simulink model "analysis_TW_UPFC"  (R2018a)
settings: Solver=FixedStepDiscrete  StartTime=0.0  StopTime=1.2  FixedStep=Ts  RelTol=1e-3
PreLoadFcn:
  | Ts=1/512/60;
undefined symbols (not defined in the file): DiscIntNeverNeededParam
libraries: powerlib x59, powerlib_meascontrol x31, simulink_extras x2, simulink x1
(part 2 of 7)

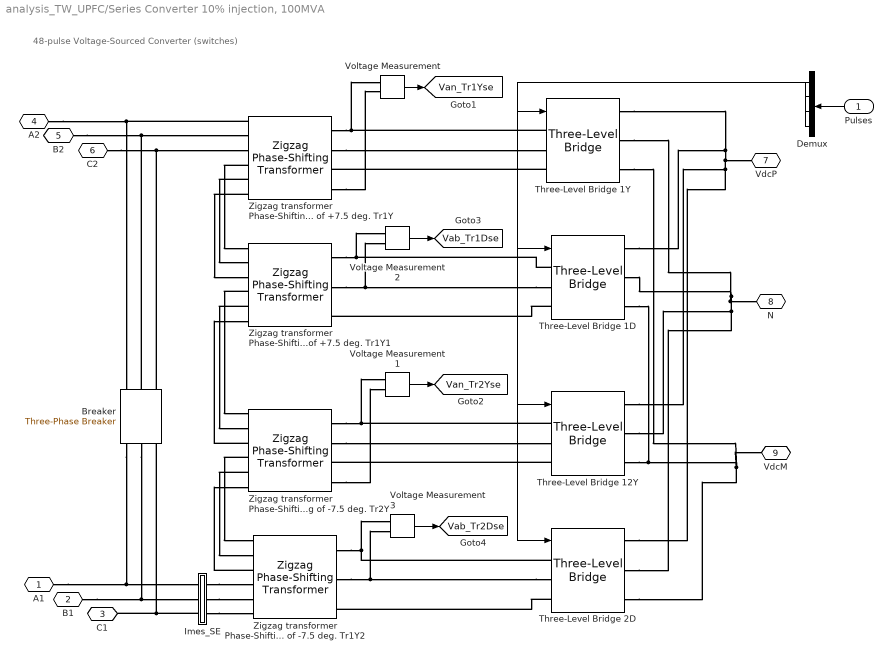
== system analysis_TW_UPFC/Series Converter 10% injection, 100MVA ==
  note: 48-pulse Voltage-Sourced Converter
      | (switches)
  Pulses : Inport  PortDimensions=48
  Breaker : powerlib/Elements/Three-Phase Breaker  InitialState=closed  SwitchA=on  SwitchB=on  SwitchC=on  SwitchTimes=[ 0]  External=off  BreakerResistance=0.0001  SnubberResistance=1e6  SnubberCapacitance=inf  Measurements=None
      settings: AttributesFormatString=\n
  Demux : Demux  Outputs=[12 12 12 12]
  Imes_SE : Subsystem
  Three-Level Bridge 12Y : powerlib/Power Electronics/Three-Level Bridge  Arms=3  SnubberResistance=1e5  SbubberCapacitance=inf  Device=GTO / Diodes  Ron=1e-4  ForwardVoltages="[  0  0  ]"  Measurements=None
      settings: SourceProductName=Simscape Power Systems  SourceProductBaseCode=PS
  Three-Level Bridge 1D : powerlib/Power Electronics/Three-Level Bridge  Arms=3  SnubberResistance=1e5  SbubberCapacitance=inf  Device=GTO / Diodes  Ron=1e-4  ForwardVoltages="[  0  0  ]"  Measurements=None
      settings: SourceProductName=Simscape Power Systems  SourceProductBaseCode=PS
  Three-Level Bridge 1Y : powerlib/Power Electronics/Three-Level Bridge  Arms=3  SnubberResistance=1e5  SbubberCapacitance=inf  Device=GTO / Diodes  Ron=1e-4  ForwardVoltages="[  0  0  ]"  Measurements=None
      settings: SourceProductName=Simscape Power Systems  SourceProductBaseCode=PS
  Three-Level Bridge 2D : powerlib/Power Electronics/Three-Level Bridge  Arms=3  SnubberResistance=1e5  SbubberCapacitance=inf  Device=GTO / Diodes  Ron=1e-4  ForwardVoltages="[  0  0  ]"  Measurements=None
      settings: SourceProductName=Simscape Power Systems  SourceProductBaseCode=PS
  Voltage Measurement{,1..3} (4 alike) : powerlib/Measurements/Voltage Measurement  Tag=PoWeRsYsTeMmEaSuReMeNt  PhasorSimulation=off  OutputType=Magnitude  PSBequivalent=0
  Zigzag transformer Phase-Shifting of +7.5 deg. Tr1Y : powerlib/Elements/Zigzag Phase-Shifting Transformer  SecondaryConnection=Yn  SetSaturation=off  SetInitialFlux=off  Measurements=None  UNITS=pu  NominalPower=[ 100e6/4 60]  PrimaryVoltage=12.5e3  SecondaryVoltage="[ 12.5e3  +7.5]"  Winding1=[ 0.05/30 0.05 ]  Winding2=[ 0.05/30 0.05 ]  Winding3=[ 0.05/30 0.05 ]  RmLm=[ 500 500 ]  Rm=500  Saturation=[ 0,0 ; 0.0024,1.2 ; 1.0,1.52 ]  InitialFluxes=[0,0,0]  MoreParameters=off  BreakLoop=off  DataType=off
      settings: AttributesFormatString=\n  SourceProductName=Simscape Power Systems  SourceProductBaseCode=PS
  Zigzag transformer Phase-Shifting of +7.5 deg. Tr1Y1 : powerlib/Elements/Zigzag Phase-Shifting Transformer  SecondaryConnection=Delta D1(-30 deg.)  SetSaturation=off  SetInitialFlux=off  Measurements=None  UNITS=pu  NominalPower=[ 100e6/4 60]  PrimaryVoltage=12.5e3  SecondaryVoltage="[ 12.5e3  +7.5]"  Winding1=[ 0.05/30 0.05 ]  Winding2=[ 0.05/30 0.05 ]  Winding3=[ 0.05/30 0.05 ]  RmLm=[ 500 500 ]  Rm=500  Saturation=[ 0,0 ; 0.0024,1.2 ; 1.0,1.52 ]  InitialFluxes=[0,0,0]  MoreParameters=off  BreakLoop=off  DataType=off
      settings: AttributesFormatString=\n  SourceProductName=Simscape Power Systems  SourceProductBaseCode=PS
  Zigzag transformer Phase-Shifting of -7.5 deg. Tr1Y2 : powerlib/Elements/Zigzag Phase-Shifting Transformer  SecondaryConnection=Delta D1(-30 deg.)  SetSaturation=off  SetInitialFlux=off  Measurements=None  UNITS=pu  NominalPower=[ 100e6/4 60]  PrimaryVoltage=12.5e3  SecondaryVoltage="[ 12.5e3  -7.5]"  Winding1=[ 0.05/30 0.05 ]  Winding2=[ 0.05/30 0.05 ]  Winding3=[ 0.05/30 0.05 ]  RmLm=[ 500 500 ]  Rm=500  Saturation=[ 0,0 ; 0.0024,1.2 ; 1.0,1.52 ]  InitialFluxes=[0,0,0]  MoreParameters=off  BreakLoop=off  DataType=off
      settings: AttributesFormatString=\n  SourceProductName=Simscape Power Systems  SourceProductBaseCode=PS
  Zigzag transformer Phase-Shifting of -7.5 deg. Tr2Y : powerlib/Elements/Zigzag Phase-Shifting Transformer  SecondaryConnection=Yn  SetSaturation=off  SetInitialFlux=off  Measurements=None  UNITS=pu  NominalPower=[ 100e6/4 60]  PrimaryVoltage=12.5e3  SecondaryVoltage="[ 12.5e3  -7.5]"  Winding1=[ 0.05/30 0.05 ]  Winding2=[ 0.05/30 0.05 ]  Winding3=[ 0.05/30 0.05 ]  RmLm=[ 500 500 ]  Rm=500  Saturation=[ 0,0 ; 0.0024,1.2 ; 1.0,1.52 ]  InitialFluxes=[0,0,0]  MoreParameters=off  BreakLoop=off  DataType=off
      settings: AttributesFormatString=\n  SourceProductName=Simscape Power Systems  SourceProductBaseCode=PS
  "A1 " : PMIOPort  Side=Left
  "B1 " : PMIOPort  Port=2  Side=Left
  C1 : PMIOPort  Port=3  Side=Left
  "A2 " : PMIOPort  Port=4  Side=Left
  "B2 " : PMIOPort  Port=5  Side=Left
  "C2 " : PMIOPort  Port=6  Side=Left
  VdcP : PMIOPort  Port=7  Side=Right
  N : PMIOPort  Port=8  Side=Right
  VdcM : PMIOPort  Port=9  Side=Right
  tag scope: Vab_Tr1Dse=global, Vab_Tr2Dse=global, Van_Tr1Yse=global, Van_Tr2Yse=global
  wires:
  Pulses/1 -> Demux/1
  Demux/4 -> Three-Level Bridge 2D/1
  Demux/3 -> Three-Level Bridge 12Y/1
  Demux/2 -> Three-Level Bridge 1D/1
  Demux/1 -> Three-Level Bridge 1Y/1
  Voltage Measurement3/1 -> [Vab_Tr2Dse]
  Voltage Measurement2/1 -> [Vab_Tr1Dse]
  Voltage Measurement1/1 -> [Van_Tr2Yse]
  Voltage Measurement/1 -> [Van_Tr1Yse]
  connections:
  Zigzag transformer Phase-Shifting of -7.5 deg. Tr2Y/RConn4 -- Voltage Measurement1/LConn2
  Zigzag transformer Phase-Shifting of +7.5 deg. Tr1Y/RConn4 -- Voltage Measurement/LConn2
  Three-Level Bridge 1Y/RConn3 -- Three-Level Bridge 1D/RConn3 -- Three-Level Bridge 12Y/RConn3 -- VdcM/RConn1 -- Three-Level Bridge 2D/RConn3
  Three-Level Bridge 12Y/RConn2 -- Three-Level Bridge 1D/RConn2 -- Three-Level Bridge 1Y/RConn2 -- N/RConn1 -- Three-Level Bridge 2D/RConn2
  Three-Level Bridge 1Y/RConn1 -- Three-Level Bridge 12Y/RConn1 -- Three-Level Bridge 2D/RConn1 -- VdcP/RConn1 -- Three-Level Bridge 1D/RConn1
  Three-Level Bridge 1D/LConn1 -- Zigzag transformer Phase-Shifting of +7.5 deg. Tr1Y1/RConn1 -- Voltage Measurement2/LConn1
  Imes_SE/RConn1 -- Zigzag transformer Phase-Shifting of -7.5 deg. Tr1Y2/LConn4
  Imes_SE/RConn2 -- Zigzag transformer Phase-Shifting of -7.5 deg. Tr1Y2/LConn5
  Imes_SE/RConn3 -- Zigzag transformer Phase-Shifting of -7.5 deg. Tr1Y2/LConn6
  "A1 "/RConn1 -- Imes_SE/LConn1 -- Breaker/RConn1
  Zigzag transformer Phase-Shifting of +7.5 deg. Tr1Y/LConn4 -- Zigzag transformer Phase-Shifting of +7.5 deg. Tr1Y1/LConn1
  Zigzag transformer Phase-Shifting of +7.5 deg. Tr1Y/LConn5 -- Zigzag transformer Phase-Shifting of +7.5 deg. Tr1Y1/LConn2
  Zigzag transformer Phase-Shifting of +7.5 deg. Tr1Y/LConn6 -- Zigzag transformer Phase-Shifting of +7.5 deg. Tr1Y1/LConn3
  Zigzag transformer Phase-Shifting of +7.5 deg. Tr1Y1/LConn4 -- Zigzag transformer Phase-Shifting of -7.5 deg. Tr2Y/LConn1
  Zigzag transformer Phase-Shifting of +7.5 deg. Tr1Y1/LConn5 -- Zigzag transformer Phase-Shifting of -7.5 deg. Tr2Y/LConn2
  Zigzag transformer Phase-Shifting of -7.5 deg. Tr2Y/LConn3 -- Zigzag transformer Phase-Shifting of +7.5 deg. Tr1Y1/LConn6
  Zigzag transformer Phase-Shifting of -7.5 deg. Tr2Y/LConn4 -- Zigzag transformer Phase-Shifting of -7.5 deg. Tr1Y2/LConn1
  Zigzag transformer Phase-Shifting of -7.5 deg. Tr2Y/LConn5 -- Zigzag transformer Phase-Shifting of -7.5 deg. Tr1Y2/LConn2
  Zigzag transformer Phase-Shifting of -7.5 deg. Tr1Y2/LConn3 -- Zigzag transformer Phase-Shifting of -7.5 deg. Tr2Y/LConn6
  Three-Level Bridge 1Y/LConn1 -- Zigzag transformer Phase-Shifting of +7.5 deg. Tr1Y/RConn1 -- Voltage Measurement/LConn1
  Three-Level Bridge 12Y/LConn1 -- Zigzag transformer Phase-Shifting of -7.5 deg. Tr2Y/RConn1 -- Voltage Measurement1/LConn1
  Three-Level Bridge 2D/LConn1 -- Zigzag transformer Phase-Shifting of -7.5 deg. Tr1Y2/RConn1 -- Voltage Measurement3/LConn1
  Imes_SE/LConn3 -- Breaker/RConn3 -- C1/RConn1
  "B1 "/RConn1 -- Imes_SE/LConn2 -- Breaker/RConn2
  Breaker/LConn3 -- Zigzag transformer Phase-Shifting of +7.5 deg. Tr1Y/LConn3 -- "C2 "/RConn1
  Breaker/LConn2 -- Zigzag transformer Phase-Shifting of +7.5 deg. Tr1Y/LConn2 -- "B2 "/RConn1
  Zigzag transformer Phase-Shifting of +7.5 deg. Tr1Y/LConn1 -- Breaker/LConn1 -- "A2 "/RConn1
  Three-Level Bridge 1Y/LConn3 -- Zigzag transformer Phase-Shifting of +7.5 deg. Tr1Y/RConn3
  Zigzag transformer Phase-Shifting of +7.5 deg. Tr1Y/RConn2 -- Three-Level Bridge 1Y/LConn2
  Three-Level Bridge 1D/LConn2 -- Zigzag transformer Phase-Shifting of +7.5 deg. Tr1Y1/RConn2 -- Voltage Measurement2/LConn2
  Three-Level Bridge 1D/LConn3 -- Zigzag transformer Phase-Shifting of +7.5 deg. Tr1Y1/RConn3
  Zigzag transformer Phase-Shifting of -7.5 deg. Tr2Y/RConn2 -- Three-Level Bridge 12Y/LConn2
  Three-Level Bridge 12Y/LConn3 -- Zigzag transformer Phase-Shifting of -7.5 deg. Tr2Y/RConn3
  Three-Level Bridge 2D/LConn2 -- Zigzag transformer Phase-Shifting of -7.5 deg. Tr1Y2/RConn2 -- Voltage Measurement3/LConn2
  Three-Level Bridge 2D/LConn3 -- Zigzag transformer Phase-Shifting of -7.5 deg. Tr1Y2/RConn3

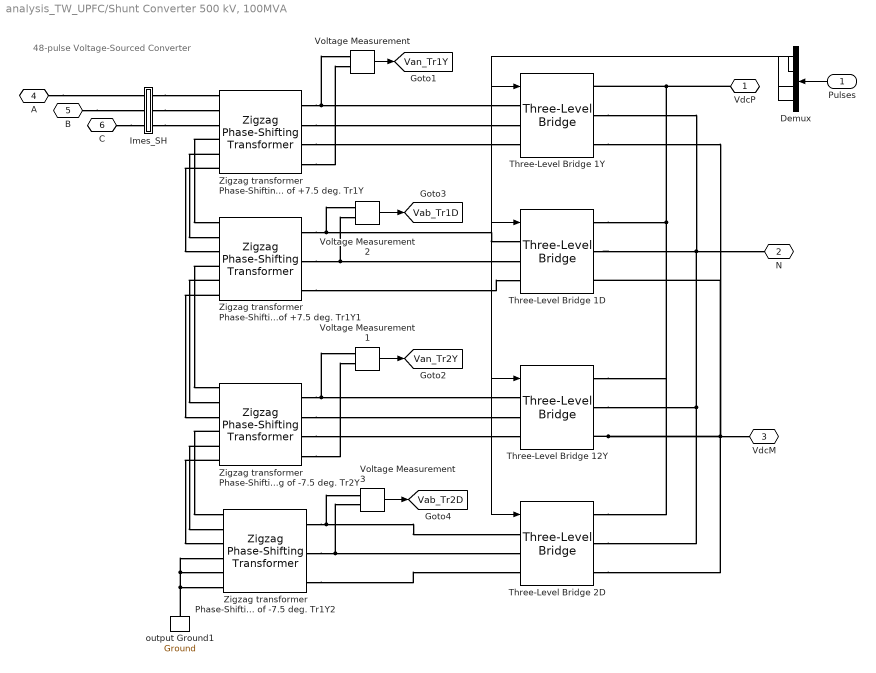
== system analysis_TW_UPFC/Shunt Converter 500 kV, 100MVA ==
  note: 48-pulse Voltage-Sourced Converter
  Pulses : Inport  PortDimensions=48
  Demux : Demux  Outputs=[12 12 12 12]
  Imes_SH : Subsystem
  Three-Level Bridge 12Y : powerlib/Power Electronics/Three-Level Bridge  Arms=3  SnubberResistance=1e5  SbubberCapacitance=inf  Device=GTO / Diodes  Ron=1e-4  ForwardVoltages="[  0  0  ]"  Measurements=None
      settings: SourceProductName=Simscape Power Systems  SourceProductBaseCode=PS
  Three-Level Bridge 1D : powerlib/Power Electronics/Three-Level Bridge  Arms=3  SnubberResistance=1e5  SbubberCapacitance=inf  Device=GTO / Diodes  Ron=1e-4  ForwardVoltages="[  0  0  ]"  Measurements=None
      settings: SourceProductName=Simscape Power Systems  SourceProductBaseCode=PS
  Three-Level Bridge 1Y : powerlib/Power Electronics/Three-Level Bridge  Arms=3  SnubberResistance=1e5  SbubberCapacitance=inf  Device=GTO / Diodes  Ron=1e-4  ForwardVoltages="[  0  0  ]"  Measurements=None
      settings: SourceProductName=Simscape Power Systems  SourceProductBaseCode=PS
  Three-Level Bridge 2D : powerlib/Power Electronics/Three-Level Bridge  Arms=3  SnubberResistance=1e5  SbubberCapacitance=inf  Device=GTO / Diodes  Ron=1e-4  ForwardVoltages="[  0  0  ]"  Measurements=None
      settings: SourceProductName=Simscape Power Systems  SourceProductBaseCode=PS
  Voltage Measurement{,1..3} (4 alike) : powerlib/Measurements/Voltage Measurement  Tag=PoWeRsYsTeMmEaSuReMeNt  PhasorSimulation=off  OutputType=Magnitude  PSBequivalent=0
  Zigzag transformer Phase-Shifting of +7.5 deg. Tr1Y : powerlib/Elements/Zigzag Phase-Shifting Transformer  SecondaryConnection=Yn  SetSaturation=off  SetInitialFlux=off  Measurements=None  UNITS=pu  NominalPower=[ 100e6/4 60]  PrimaryVoltage=500e3/4  SecondaryVoltage="[ 15e3  +7.5]"  Winding1=[ 0.05/30 0.05 ]  Winding2=[ 0.05/30 0.05 ]  Winding3=[ 0.05/30 0.05 ]  RmLm=[ 500 500 ]  Rm=500  Saturation=[ 0,0 ; 0.0024,1.2 ; 1.0,1.52 ]  InitialFluxes=[0,0,0]  MoreParameters=off  BreakLoop=off  DataType=off
      settings: AttributesFormatString=\n  SourceProductName=Simscape Power Systems  SourceProductBaseCode=PS
  Zigzag transformer Phase-Shifting of +7.5 deg. Tr1Y1 : powerlib/Elements/Zigzag Phase-Shifting Transformer  SecondaryConnection=Delta D1(-30 deg.)  SetSaturation=off  SetInitialFlux=off  Measurements=None  UNITS=pu  NominalPower=[ 100e6/4 60]  PrimaryVoltage=500e3/4  SecondaryVoltage="[ 15e3  +7.5]"  Winding1=[ 0.05/30 0.05 ]  Winding2=[ 0.05/30 0.05 ]  Winding3=[ 0.05/30 0.05 ]  RmLm=[ 500 500 ]  Rm=500  Saturation=[ 0,0 ; 0.0024,1.2 ; 1.0,1.52 ]  InitialFluxes=[0,0,0]  MoreParameters=off  BreakLoop=off  DataType=off
      settings: AttributesFormatString=\n  SourceProductName=Simscape Power Systems  SourceProductBaseCode=PS
  Zigzag transformer Phase-Shifting of -7.5 deg. Tr1Y2 : powerlib/Elements/Zigzag Phase-Shifting Transformer  SecondaryConnection=Delta D1(-30 deg.)  SetSaturation=off  SetInitialFlux=off  Measurements=None  UNITS=pu  NominalPower=[ 100e6/4 60]  PrimaryVoltage=500e3/4  SecondaryVoltage="[ 15e3  -7.5]"  Winding1=[ 0.05/30 0.05 ]  Winding2=[ 0.05/30 0.05 ]  Winding3=[ 0.05/30 0.05 ]  RmLm=[ 500 500 ]  Rm=500  Saturation=[ 0,0 ; 0.0024,1.2 ; 1.0,1.52 ]  InitialFluxes=[0,0,0]  MoreParameters=off  BreakLoop=off  DataType=off
      settings: AttributesFormatString=\n  SourceProductName=Simscape Power Systems  SourceProductBaseCode=PS
  Zigzag transformer Phase-Shifting of -7.5 deg. Tr2Y : powerlib/Elements/Zigzag Phase-Shifting Transformer  SecondaryConnection=Yn  SetSaturation=off  SetInitialFlux=off  Measurements=None  UNITS=pu  NominalPower=[ 100e6/4 60]  PrimaryVoltage=500e3/4  SecondaryVoltage="[ 15e3  -7.5]"  Winding1=[ 0.05/30 0.05 ]  Winding2=[ 0.05/30 0.05 ]  Winding3=[ 0.05/30 0.05 ]  RmLm=[ 500 500 ]  Rm=500  Saturation=[ 0,0 ; 0.0024,1.2 ; 1.0,1.52 ]  InitialFluxes=[0,0,0]  MoreParameters=off  BreakLoop=off  DataType=off
      settings: AttributesFormatString=\n  SourceProductName=Simscape Power Systems  SourceProductBaseCode=PS
  output Ground1 : powerlib/Elements/Ground  LConnTagsString=a  RConnTagsString=__newr0
  VdcP : PMIOPort  Side=Right
  N : PMIOPort  Port=2  Side=Right
  VdcM : PMIOPort  Port=3  Side=Right
  A : PMIOPort  Port=4  Side=Left
  B : PMIOPort  Port=5  Side=Left
  C : PMIOPort  Port=6  Side=Left
  tag scope: Vab_Tr1D=global, Vab_Tr2D=global, Van_Tr1Y=global, Van_Tr2Y=global
  wires:
  Pulses/1 -> Demux/1
  Voltage Measurement/1 -> [Van_Tr1Y]
  Voltage Measurement1/1 -> [Van_Tr2Y]
  Voltage Measurement2/1 -> [Vab_Tr1D]
  Voltage Measurement3/1 -> [Vab_Tr2D]
  Demux/1 -> Three-Level Bridge 1Y/1
  Demux/2 -> Three-Level Bridge 1D/1
  Demux/3 -> Three-Level Bridge 12Y/1
  Demux/4 -> Three-Level Bridge 2D/1
  connections:
  VdcP/RConn1 -- Three-Level Bridge 12Y/RConn1 -- Three-Level Bridge 2D/RConn1 -- Three-Level Bridge 1D/RConn1 -- Three-Level Bridge 1Y/RConn1
  Zigzag transformer Phase-Shifting of +7.5 deg. Tr1Y/RConn2 -- Three-Level Bridge 1Y/LConn2
  Zigzag transformer Phase-Shifting of +7.5 deg. Tr1Y/RConn3 -- Three-Level Bridge 1Y/LConn3
  Zigzag transformer Phase-Shifting of -7.5 deg. Tr2Y/RConn2 -- Three-Level Bridge 12Y/LConn2
  Zigzag transformer Phase-Shifting of -7.5 deg. Tr2Y/RConn3 -- Three-Level Bridge 12Y/LConn3
  Zigzag transformer Phase-Shifting of +7.5 deg. Tr1Y/RConn4 -- Voltage Measurement/LConn2
  Zigzag transformer Phase-Shifting of -7.5 deg. Tr2Y/RConn4 -- Voltage Measurement1/LConn2
  Imes_SH/RConn1 -- Zigzag transformer Phase-Shifting of +7.5 deg. Tr1Y/LConn1
  Imes_SH/RConn2 -- Zigzag transformer Phase-Shifting of +7.5 deg. Tr1Y/LConn2
  Imes_SH/RConn3 -- Zigzag transformer Phase-Shifting of +7.5 deg. Tr1Y/LConn3
  B/RConn1 -- Imes_SH/LConn2
  A/RConn1 -- Imes_SH/LConn1
  C/RConn1 -- Imes_SH/LConn3
  Zigzag transformer Phase-Shifting of +7.5 deg. Tr1Y/LConn4 -- Zigzag transformer Phase-Shifting of +7.5 deg. Tr1Y1/LConn1
  Zigzag transformer Phase-Shifting of +7.5 deg. Tr1Y/LConn5 -- Zigzag transformer Phase-Shifting of +7.5 deg. Tr1Y1/LConn2
  Zigzag transformer Phase-Shifting of +7.5 deg. Tr1Y/LConn6 -- Zigzag transformer Phase-Shifting of +7.5 deg. Tr1Y1/LConn3
  Zigzag transformer Phase-Shifting of +7.5 deg. Tr1Y1/LConn4 -- Zigzag transformer Phase-Shifting of -7.5 deg. Tr2Y/LConn1
  Zigzag transformer Phase-Shifting of +7.5 deg. Tr1Y1/LConn5 -- Zigzag transformer Phase-Shifting of -7.5 deg. Tr2Y/LConn2
  Zigzag transformer Phase-Shifting of +7.5 deg. Tr1Y1/LConn6 -- Zigzag transformer Phase-Shifting of -7.5 deg. Tr2Y/LConn3
  Zigzag transformer Phase-Shifting of -7.5 deg. Tr2Y/LConn4 -- Zigzag transformer Phase-Shifting of -7.5 deg. Tr1Y2/LConn1
  Zigzag transformer Phase-Shifting of -7.5 deg. Tr2Y/LConn5 -- Zigzag transformer Phase-Shifting of -7.5 deg. Tr1Y2/LConn2
  Zigzag transformer Phase-Shifting of -7.5 deg. Tr2Y/LConn6 -- Zigzag transformer Phase-Shifting of -7.5 deg. Tr1Y2/LConn3
  output Ground1/LConn1 -- Zigzag transformer Phase-Shifting of -7.5 deg. Tr1Y2/LConn4 -- Zigzag transformer Phase-Shifting of -7.5 deg. Tr1Y2/LConn5 -- Zigzag transformer Phase-Shifting of -7.5 deg. Tr1Y2/LConn6
  Three-Level Bridge 12Y/RConn3 -- Three-Level Bridge 1Y/RConn3 -- Three-Level Bridge 1D/RConn3 -- Three-Level Bridge 2D/RConn3 -- VdcM/RConn1
  Zigzag transformer Phase-Shifting of +7.5 deg. Tr1Y1/RConn1 -- Three-Level Bridge 1D/LConn1 -- Voltage Measurement2/LConn1
  Zigzag transformer Phase-Shifting of +7.5 deg. Tr1Y1/RConn2 -- Three-Level Bridge 1D/LConn2 -- Voltage Measurement2/LConn2
  Zigzag transformer Phase-Shifting of +7.5 deg. Tr1Y1/RConn3 -- Three-Level Bridge 1D/LConn3
  Three-Level Bridge 12Y/RConn2 -- Three-Level Bridge 1D/RConn2 -- N/RConn1 -- Three-Level Bridge 1Y/RConn2 -- Three-Level Bridge 2D/RConn2
  Zigzag transformer Phase-Shifting of +7.5 deg. Tr1Y/RConn1 -- Three-Level Bridge 1Y/LConn1 -- Voltage Measurement/LConn1
  Zigzag transformer Phase-Shifting of -7.5 deg. Tr2Y/RConn1 -- Three-Level Bridge 12Y/LConn1 -- Voltage Measurement1/LConn1
  Zigzag transformer Phase-Shifting of -7.5 deg. Tr1Y2/RConn1 -- Three-Level Bridge 2D/LConn1 -- Voltage Measurement3/LConn1
  Zigzag transformer Phase-Shifting of -7.5 deg. Tr1Y2/RConn2 -- Three-Level Bridge 2D/LConn2 -- Voltage Measurement3/LConn2
  Zigzag transformer Phase-Shifting of -7.5 deg. Tr1Y2/RConn3 -- Three-Level Bridge 2D/LConn3

== system analysis_TW_UPFC/Subsystem ==
  Sw1 : powerlib/Power Electronics/Ideal Switch  Ron=0.0001  Lon=0  IC=0  Rs=inf  Cs=0  Measurements=off
      settings: AttributesFormatString=\n
  Sw2 : powerlib/Power Electronics/Ideal Switch  Ron=0.0001  Lon=0  IC=0  Rs=inf  Cs=0  Measurements=off
      settings: AttributesFormatString=\n
  "VdcP " : PMIOPort  Side=Left
  "N " : PMIOPort  Port=2  Side=Left
  "VdcM " : PMIOPort  Port=3  Side=Left
  " VdcP" : PMIOPort  Port=4  Side=Right
  " N" : PMIOPort  Port=5  Side=Right
  " VdcM" : PMIOPort  Port=6  Side=Right
  wires:
  [Sw_On] -> Sw1/1, Sw2/1
  connections:
  " VdcP"/RConn1 -- Sw1/RConn1
  "VdcP "/RConn1 -- Sw1/LConn1
  " VdcM"/RConn1 -- Sw2/RConn1
  "VdcM "/RConn1 -- Sw2/LConn1
  "N "/RConn1 -- " N"/RConn1

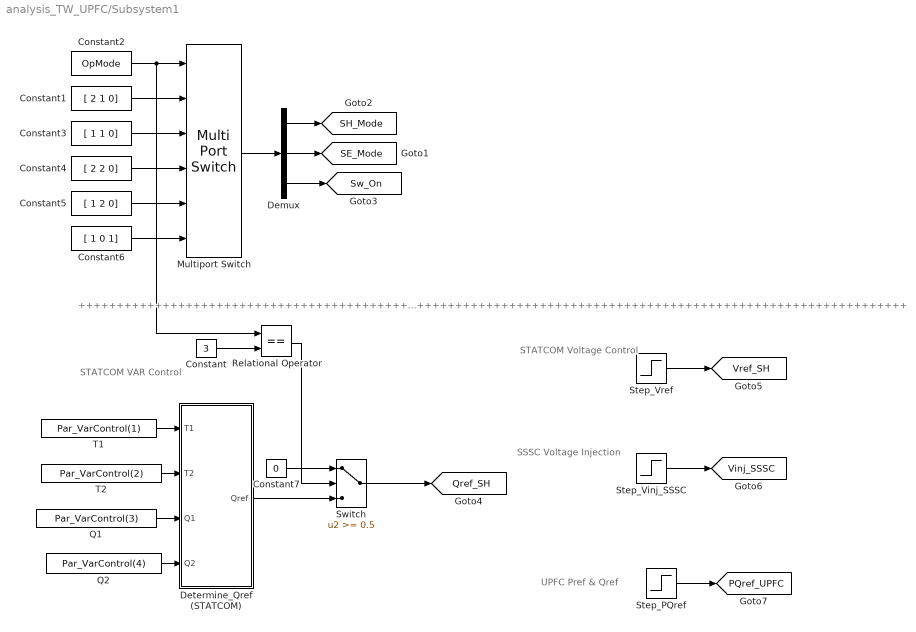
== system analysis_TW_UPFC/Subsystem1 ==
  note: +++++++++++++++++++++++++++++++++++++++++++++++++++++++++++++++++++++++++++++++++++++++++++++++++++++++++++++++++++
  note: STATCOM
      | VAR Control
  note: STATCOM
      | Voltage Control
  note: SSSC
      | Voltage Injection
  note: UPFC
      | Pref & Qref
  Constant : Constant  Value=3
  Constant1 : Constant  Value=[ 2 1 0]
  Constant2 : Constant  Value=OpMode
  Constant3 : Constant  Value=[ 1 1 0]
  Constant4 : Constant  Value=[ 2 2 0]
  Constant5 : Constant  Value=[ 1 2 0]
  Constant6 : Constant  Value=[ 1 0 1]
  Constant7 : Constant  Value=0
  Demux : Demux  Outputs=3
  Determine_Qref (STATCOM) : Subsystem
  Multiport Switch : MultiPortSwitch  Inputs=5  SaturateOnIntegerOverflow=on
  Q1 : Constant  Value=Par_VarControl(3)
  Q2 : Constant  Value=Par_VarControl(4)
  Relational Operator : RelationalOperator  Operator===  RndMeth=Nearest
  Step_PQref : Step  Time=[Par_UPFC_Pref(3) Par_UPFC_Qref(3) ]  Before=[Par_UPFC_Pref(1) Par_UPFC_Qref(1) ]  After=[Par_UPFC_Pref(2) Par_UPFC_Qref(2) ]  SampleTime=0
  Step_Vinj_SSSC : Step  Time=Par_SSSC(3)  Before=Par_SSSC(1)  After=Par_SSSC(2)  SampleTime=0
  Step_Vref : Step  Time=Par_Vref(3)  Before=Par_Vref(1)  After=Par_Vref(2)  SampleTime=0
  Switch : Switch  Threshold=0.5  SaturateOnIntegerOverflow=on
  T1 : Constant  Value=Par_VarControl(1)
  T2 : Constant  Value=Par_VarControl(2)
  tag scope: PQref_UPFC=global, Qref_SH=global, SE_Mode=global, SH_Mode=global, Sw_On=global, Vinj_SSSC=global, Vref_SH=global
  wires:
  Constant2/1 -> Multiport Switch/1, Relational Operator/1
  Multiport Switch/1 -> Demux/1
  Demux/1 -> [SH_Mode]
  Demux/2 -> [SE_Mode]
  Demux/3 -> [Sw_On]
  Constant1/1 -> Multiport Switch/2
  Constant6/1 -> Multiport Switch/6
  Constant5/1 -> Multiport Switch/5
  Constant3/1 -> Multiport Switch/3
  Constant4/1 -> Multiport Switch/4
  T1/1 -> Determine_Qref (STATCOM)/1(T1)
  T2/1 -> Determine_Qref (STATCOM)/2(T2)
  Q1/1 -> Determine_Qref (STATCOM)/3(Q1)
  Q2/1 -> Determine_Qref (STATCOM)/4(Q2)
  Determine_Qref (STATCOM)/1(Qref) -> Switch/3
  Switch/1 -> [Qref_SH]
  Constant/1 -> Relational Operator/2
  Relational Operator/1 -> Switch/2
  Constant7/1 -> Switch/1
  Step_Vref/1 -> [Vref_SH]
  Step_PQref/1 -> [PQref_UPFC]
  Step_Vinj_SSSC/1 -> [Vinj_SSSC]

== system analysis_TW_UPFC/Subsystem2 ==

== system analysis_TW_UPFC/Subsystem4 ==
  Data Acquisition : Subsystem
  Mux : Mux  Inputs=2
  SSSC : Scope  NumInputPorts=6
  STATCOM : Scope  NumInputPorts=4
  Selector : Selector  InputPortWidth=3  IndexOptions=Index vector (dialog)  Indices=2  OutputSizes=1
  Selector1 : Selector  InputPortWidth=3  IndexOptions=Index vector (dialog)  Indices=2  OutputSizes=1
  Selector2 : Selector  InputPortWidth=2  IndexOptions=Index vector (dialog)  Indices=1  OutputSizes=1
  UPFC : Scope  NumInputPorts=4
  tag scope: Display_PQ=global, Display_V1=global
  wires:
  Data Acquisition/1(VsVpI_SH) -> STATCOM/1  "Vs Vp Ip (pu)"
  Data Acquisition/2(Vdc_SH) -> STATCOM/2  "Vdc (V)"
  Data Acquisition/3(Q_Qref_SH) -> STATCOM/3  "Q Qref (pu)"
  Data Acquisition/4(VmeasVref_SH) -> STATCOM/4, Selector2/1  "Vmeas Vref (pu)"
  Data Acquisition/6(Iabc_SE) -> SSSC/2  "Iabc (pu)"
  Data Acquisition/5(Vinj_SE) -> SSSC/1  "Vinj (pu)"
  Data Acquisition/7(Vmeas_Vref_SSSC) -> SSSC/3  "Mag_Vinj  / Vref (pu)"
  Data Acquisition/8(Vdc_SE) -> SSSC/4  "Vdc"
  Data Acquisition/9(P_L123) -> UPFC/3, SSSC/5, Selector/1  "P L1 L2 L3 (MW)"
  Data Acquisition/10(Q_L123) -> UPFC/4, SSSC/6, Selector1/1  "Q L1 L2 L3 (Mvar)"
  Data Acquisition/11(P_Pref_SE) -> UPFC/1  "P Pref (pu)"
  Data Acquisition/12(Q_Qref_SE) -> UPFC/2  "Q Qref (pu)"
  Selector/1 -> Mux/1
  Selector1/1 -> Mux/2
  Mux/1 -> [Display_PQ]
  Selector2/1 -> [Display_V1]

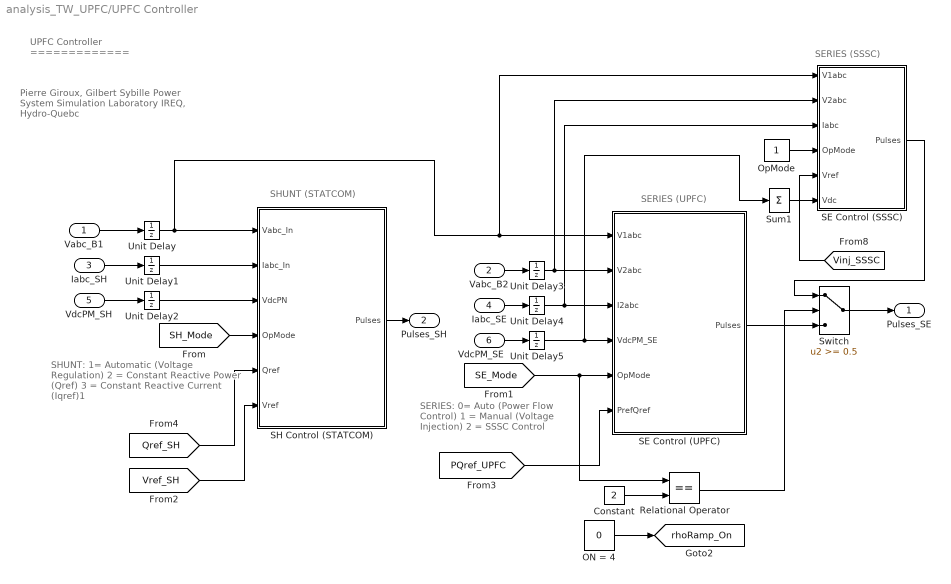
== system analysis_TW_UPFC/UPFC Controller ==
  note: Pierre Giroux, Gilbert Sybille
      | Power System Simulation Laboratory
      | IREQ, Hydro-Quebc
  note: SHUNT (STATCOM)
  note: SERIES (UPFC)
  note: UPFC Controller
      | =============
  note: SHUNT:
      | 1= Automatic (Voltage Regulation)
      | 2 = Constant Reactive Power (Qref)
      | 3 = Constant Reactive Current (Iqref)1
  note: SERIES:
      | 0= Auto (Power Flow Control)
      | 1 = Manual (Voltage Injection)
      | 2 = SSSC Control
  note: SERIES (SSSC)
  Vabc_B1 : Inport  PortDimensions=3
  Vabc_B2 : Inport  Port=2  PortDimensions=3
  "Iabc_SH " : Inport  Port=3  PortDimensions=3
  Iabc_SE : Inport  Port=4  PortDimensions=3
  "VdcPM_SH " : Inport  Port=5  PortDimensions=2
  VdcPM_SE : Inport  Port=6  PortDimensions=2
  Constant : Constant  Value=2
  ON = 4 : Constant  Value=0
  OpMode : Constant
  Relational Operator : RelationalOperator  Operator===  RndMeth=Nearest
  SE Control (SSSC) : Subsystem
  SE Control (UPFC) : Subsystem  mask(Injection Voltage Control){PQref=[8.7 -0.6], Vref_Inj=[0 0], ParK_Vseries=[0.045 1.5*4], Ts=Ts}
      mask prompts: PQref "Reference active and reactive power [ Pref  Qref ] (pu/100MVA):"; Vref_Inj "Manual Voltage Injection: [ Mag(pu)  rho(deg.) ]"; ParK_Vseries "Regulator gain [Kp  Ki ]"; Ts "Sample time:"
      mask init:
      | Kp_Vseries=ParK_Vseries(1);
      | Ki_Vseries=ParK_Vseries(2);
      | Pref=PQref(1);
      | Qref=PQref(2);
      | MagInj=Vref_Inj(1);
      | rhoInj=Vref_Inj(2);
  SH Control (STATCOM) : Subsystem  mask(STATCOM Controller){Vref=1.00, Droop=0.01, Qref1=0, Iqref1=0, ParK_V=[12 3000]*3, ParK_I=[5 40], Ts=Ts}
      mask prompts: Vref "Automatic mode: Voltage setpoint (Vref in pu)"; Droop "Droop (pu/100 MVA):"; Qref1 "Reactive power setpoint (Qref in pu)"; Iqref1 "Reactive Current setpoint (Iqref in pu):"; ParK_V "Voltage regulator gains: [ Kp  Ki ]"; ParK_I "Iq regulator gains: [ Kp  Ki ]"; Ts "Sample time:"
      mask init:
      | Kp_I=ParK_I(1);
      | Ki_I=ParK_I(2);
      | Kp_V=ParK_V(1);
      | Ki_V=ParK_V(2);
  Sum1 : Sum  Inputs=1  SaturateOnIntegerOverflow=on  InputSameDT=on  OutDataTypeStr=Inherit: Same as first input
  Switch : Switch  Threshold=0.5  SaturateOnIntegerOverflow=on
  Unit Delay{,1..5} (6 alike) : UnitDelay  SampleTime=Ts
  Pulses_SE : Outport
  Pulses_SH : Outport  Port=2
  tag scope: rhoRamp_On=global
  wires:
  "Iabc_SH "/1 -> Unit Delay1/1
  "VdcPM_SH "/1 -> Unit Delay2/1
  Vabc_B1/1 -> Unit Delay/1
  SH Control (STATCOM)/1(Pulses) -> Pulses_SH/1
  Iabc_SE/1 -> Unit Delay4/1
  Vabc_B2/1 -> Unit Delay3/1
  VdcPM_SE/1 -> Unit Delay5/1
  Unit Delay/1 -> SH Control (STATCOM)/1(Vabc_In), SE Control (UPFC)/1(V1abc), SE Control (SSSC)/1(V1abc)
  Unit Delay1/1 -> SH Control (STATCOM)/2(Iabc_In)
  Unit Delay2/1 -> SH Control (STATCOM)/3(VdcPN)
  Unit Delay3/1 -> SE Control (UPFC)/2(V2abc), SE Control (SSSC)/2(V2abc)
  Unit Delay4/1 -> SE Control (UPFC)/3(I2abc), SE Control (SSSC)/3(Iabc)
  Unit Delay5/1 -> SE Control (UPFC)/4(VdcPM_SE), Sum1/1
  ON = 4/1 -> [rhoRamp_On]
  [SE_Mode] -> SE Control (UPFC)/5(OpMode), Relational Operator/1
  OpMode/1 -> SE Control (SSSC)/4(OpMode)
  [SH_Mode] -> SH Control (STATCOM)/4(OpMode)
  Sum1/1 -> SE Control (SSSC)/6(Vdc)
  Constant/1 -> Relational Operator/2
  [Vref_SH] -> SH Control (STATCOM)/6(Vref)
  [PQref_UPFC] -> SE Control (UPFC)/6(PrefQref)
  [Vinj_SSSC] -> SE Control (SSSC)/5(Vref)
  [Qref_SH] -> SH Control (STATCOM)/5(Qref)
  SE Control (UPFC)/1(Pulses) -> Switch/3
  Switch/1 -> Pulses_SE/1
  SE Control (SSSC)/1(Pulses) -> Switch/1
  Relational Operator/1 -> Switch/2

== system analysis_TW_UPFC/info ==

== system analysis_TW_UPFC/Series Converter 10% injection, 100MVA/Imes_SE ==
  A->pu : Gain  Gain=500e3*sqrt(3)/100e6/sqrt(2)  SaturateOnIntegerOverflow=on  OutDataTypeStr=Inherit: Same as input  ParamDataTypeStr=Inherit: Same as input
  Current Measurement : powerlib/Measurements/Current Measurement  Tag=PoWeRsYsTeMmEaSuReMeNt  PhasorSimulation=off  OutputType=Magnitude  PSBequivalent=0
  Current Measurement1 : powerlib/Measurements/Current Measurement  Tag=PoWeRsYsTeMmEaSuReMeNt  PhasorSimulation=off  OutputType=Magnitude  PSBequivalent=0
  Current Measurement2 : powerlib/Measurements/Current Measurement  Tag=PoWeRsYsTeMmEaSuReMeNt  PhasorSimulation=off  OutputType=Magnitude  PSBequivalent=0
  Mux : Mux  Inputs=3
  "A " : PMIOPort  Side=Left
  "B " : PMIOPort  Port=2  Side=Left
  "C " : PMIOPort  Port=3  Side=Left
  " A" : PMIOPort  Port=4  Side=Right
  " B" : PMIOPort  Port=5  Side=Right
  " C" : PMIOPort  Port=6  Side=Right
  tag scope: Iabc_SE=global
  wires:
  Mux/1 -> A->pu/1
  A->pu/1 -> [Iabc_SE]
  Current Measurement/1 -> Mux/1
  Current Measurement2/1 -> Mux/3
  Current Measurement1/1 -> Mux/2
  connections:
  "A "/RConn1 -- Current Measurement/LConn1
  Current Measurement/RConn1 -- " A"/RConn1
  "B "/RConn1 -- Current Measurement1/LConn1
  Current Measurement1/RConn1 -- " B"/RConn1
  "C "/RConn1 -- Current Measurement2/LConn1
  Current Measurement2/RConn1 -- " C"/RConn1

== system analysis_TW_UPFC/Shunt Converter 500 kV, 100MVA/Imes_SH ==
  A->pu : Gain  Gain=500e3*sqrt(3)/100e6/sqrt(2)  SaturateOnIntegerOverflow=on  OutDataTypeStr=Inherit: Same as input  ParamDataTypeStr=Inherit: Same as input
  Current Measurement : powerlib/Measurements/Current Measurement  Tag=PoWeRsYsTeMmEaSuReMeNt  PhasorSimulation=off  OutputType=Magnitude  PSBequivalent=0
  Current Measurement1 : powerlib/Measurements/Current Measurement  Tag=PoWeRsYsTeMmEaSuReMeNt  PhasorSimulation=off  OutputType=Magnitude  PSBequivalent=0
  Current Measurement2 : powerlib/Measurements/Current Measurement  Tag=PoWeRsYsTeMmEaSuReMeNt  PhasorSimulation=off  OutputType=Magnitude  PSBequivalent=0
  Mux : Mux  Inputs=3
  "A " : PMIOPort  Side=Left
  "B " : PMIOPort  Port=2  Side=Left
  "C " : PMIOPort  Port=3  Side=Left
  " A" : PMIOPort  Port=4  Side=Right
  " B" : PMIOPort  Port=5  Side=Right
  " C" : PMIOPort  Port=6  Side=Right
  tag scope: Iabc_SH=global
  wires:
  Mux/1 -> A->pu/1
  A->pu/1 -> [Iabc_SH]
  Current Measurement/1 -> Mux/1
  Current Measurement2/1 -> Mux/3
  Current Measurement1/1 -> Mux/2
  connections:
  "A "/RConn1 -- Current Measurement/LConn1
  Current Measurement/RConn1 -- " A"/RConn1
  "B "/RConn1 -- Current Measurement1/LConn1
  Current Measurement1/RConn1 -- " B"/RConn1
  "C "/RConn1 -- Current Measurement2/LConn1
  Current Measurement2/RConn1 -- " C"/RConn1

== system analysis_TW_UPFC/Subsystem1/Determine_Qref (STATCOM) ==
  T1 : Inport
  T2 : Inport  Port=2
  Q1 : Inport  Port=3
  Q2 : Inport  Port=4
  Constant : Constant  Value=0
  Constant1 : Constant
  Digital Clock : DigitalClock  SampleTime=Ts
  Multiport Switch : MultiPortSwitch  SaturateOnIntegerOverflow=on
  Relational Operator : RelationalOperator  Operator=>  RndMeth=Nearest
  Relational Operator1 : RelationalOperator  Operator=>  RndMeth=Nearest
  Sum : Sum  Inputs=+++  SaturateOnIntegerOverflow=on
  Qref : Outport
  wires:
  Sum/1 -> Multiport Switch/1
  Q2/1 -> Multiport Switch/4
  Q1/1 -> Multiport Switch/3
  Multiport Switch/1 -> Qref/1
  Constant1/1 -> Sum/1
  Relational Operator1/1 -> Sum/3
  Relational Operator/1 -> Sum/2
  Constant/1 -> Multiport Switch/2
  T2/1 -> Relational Operator1/2
  T1/1 -> Relational Operator/2
  Digital Clock/1 -> Relational Operator1/1, Relational Operator/1

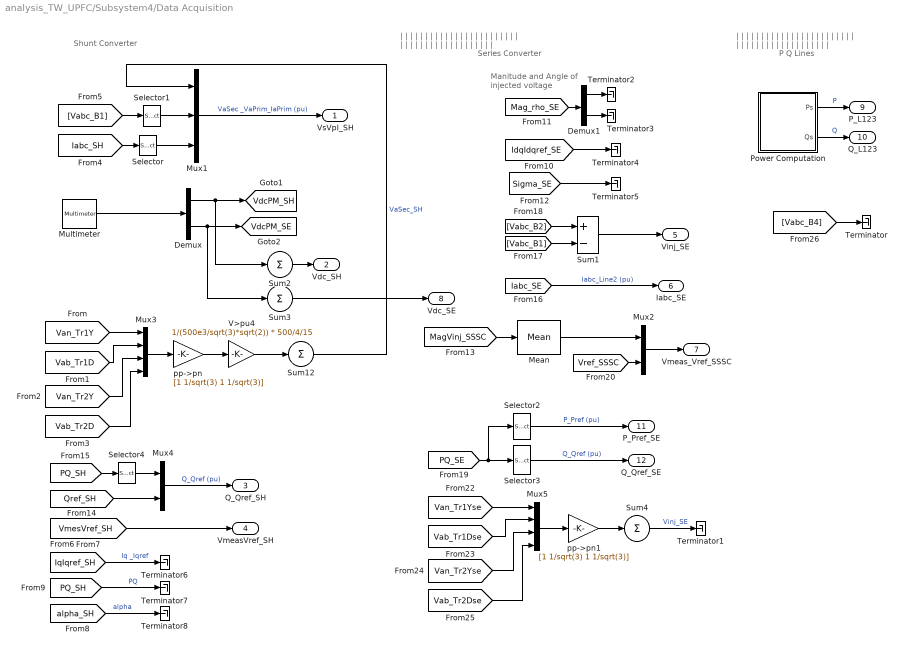
== system analysis_TW_UPFC/Subsystem4/Data Acquisition ==
  note: |
      | |
      | |
      | |
      | |
      | |
      | |
      | |
      | |
      | |
      | |
      | |
      | |
      | |
      | |
      | |
      | |
      | |
      | |
      | |
      | |
      | |
      | |
      | |
      | |
      | |
      | |
      | |
      | |
      | |
      | |
      | |
      | |
      | |
      | |
      | |
      | |
      | |
      | |
      | |
      | |
      | |
      | |
  note: Shunt Converter
  note: Series Converter
  note: |
      | |
      | |
      | |
      | |
      | |
      | |
      | |
      | |
      | |
      | |
      | |
      | |
      | |
      | |
      | |
      | |
      | |
      | |
      | |
      | |
      | |
      | |
      | |
      | |
      | |
      | |
      | |
      | |
      | |
      | |
      | |
      | |
      | |
      | |
      | |
      | |
      | |
      | |
      | |
      | |
      | |
      | |
  note: P Q Lines
  note: Manitude and Angle
      | of injected voltage
  Demux : Demux  Outputs=[2 2]
  Demux1 : Demux  Outputs=2
  Mean : powerlib_meascontrol/Measurements/Mean  Freq=60  Vinit=0  Ts=Ts
  Multimeter : powerlib/Measurements/Multimeter  Tag=PoWeRsYsTeMmEaSuReMeNt  PhasorSimulation=off  OutputType=Magnitude  sel=[4 2 3 1]  L=4  Gain=[1 1 1 1]  yselected={'Ub: Cp_SH','Ub: Cm_SH','Ub: Cp_SE','Ub: Cm_SE'};  PSBOutputType=1  PSBequivalent=0  AxesSetting=[0,0.1,-100,100]  Display=0  SavedBlockNames={}
      settings: AttributesFormatString=\n
  Mux1 : Mux  Inputs=3
  Mux2 : Mux  Inputs=2
  Mux3 : Mux
  Mux4 : Mux  Inputs=2
  Mux5 : Mux
  Power Computation : Subsystem
  Selector : Selector  InputPortWidth=3  IndexOptions=Index vector (dialog)  Indices=1  OutputSizes=1
  Selector1 : Selector  InputPortWidth=3  IndexOptions=Index vector (dialog)  Indices=1  OutputSizes=1
  Selector2 : Selector  InputPortWidth=4  IndexOptions=Index vector (dialog)  Indices=[1 3]  OutputSizes=1
  Selector3 : Selector  InputPortWidth=4  IndexOptions=Index vector (dialog)  Indices=[2 4]  OutputSizes=1
  Selector4 : Selector  InputPortWidth=2  IndexOptions=Index vector (dialog)  Indices=2  OutputSizes=1
  Sum1 : Sum  Inputs=+-  SaturateOnIntegerOverflow=on  InputSameDT=on  OutDataTypeStr=Inherit: Same as first input
  Sum{2..4,12} (4 alike) : Sum  Inputs=1  SaturateOnIntegerOverflow=on  InputSameDT=on  OutDataTypeStr=Inherit: Same as first input
  Terminator{,1..8} (9 alike) : Terminator
  V>pu4 : Gain  Gain=1/(500e3/sqrt(3)*sqrt(2)) * 500/4/15  SaturateOnIntegerOverflow=on  OutDataTypeStr=Inherit: Same as input  ParamDataTypeStr=Inherit: Same as input
  pp->pn : Gain  Gain=[1 1/sqrt(3) 1 1/sqrt(3)]  SaturateOnIntegerOverflow=on  OutDataTypeStr=Inherit: Same as input  ParamDataTypeStr=Inherit: Same as input
  pp->pn1 : Gain  Gain=[1 1/sqrt(3) 1 1/sqrt(3)]  SaturateOnIntegerOverflow=on  OutDataTypeStr=Inherit: Same as input  ParamDataTypeStr=Inherit: Same as input
  VsVpI_SH : Outport
  Vdc_SH : Outport  Port=2
  Q_Qref_SH : Outport  Port=3
  VmeasVref_SH : Outport  Port=4
  Vinj_SE : Outport  Port=5
  Iabc_SE : Outport  Port=6
  Vmeas_Vref_SSSC : Outport  Port=7
  Vdc_SE : Outport  Port=8
  P_L123 : Outport  Port=9
  Q_L123 : Outport  Port=10
  P_Pref_SE : Outport  Port=11
  Q_Qref_SE : Outport  Port=12
  tag scope: VdcPM_SE=global, VdcPM_SH=global
  wires:
  [Vref_SSSC] -> Mux2/2
  Mux2/1 -> Vmeas_Vref_SSSC/1
  [alpha_SH] -> Terminator8/1  "alpha"
  [PQ_SH] -> Terminator7/1  "PQ"
  [IqIqref_SH] -> Terminator6/1  "Iq _Iqref"
  [VmesVref_SH] -> VmeasVref_SH/1
  Selector3/1 -> Q_Qref_SE/1  "Q_Qref (pu)"
  [Sigma_SE] -> Terminator5/1
  [IdqIdqref_SE] -> Terminator4/1
  Demux1/2 -> Terminator3/1
  Demux1/1 -> Terminator2/1
  Sum4/1 -> Terminator1/1  "Vinj_SE"
  [Vabc_B4] -> Terminator/1
  [Iabc_SE] -> Iabc_SE/1  "Iabc_Line2 (pu)"
  Sum1/1 -> Vinj_SE/1
  Power Computation/2(Qs) -> Q_L123/1  "Q"
  Power Computation/1(Ps) -> P_L123/1  "P"
  [PQ_SE] -> Selector2/1, Selector3/1
  [Vabc_B1] -> Sum1/2
  [Vabc_B2] -> Sum1/1
  Selector2/1 -> P_Pref_SE/1  "P_Pref (pu)"
  [PQ_SH] -> Selector4/1
  Mux4/1 -> Q_Qref_SH/1  "Q_Qref (pu)"
  Selector4/1 -> Mux4/1
  [Qref_SH] -> Mux4/2
  V>pu4/1 -> Sum12/1
  pp->pn/1 -> V>pu4/1
  Mux3/1 -> pp->pn/1
  [Van_Tr1Y] -> Mux3/1
  [Vab_Tr1D] -> Mux3/2
  [Van_Tr2Y] -> Mux3/3
  [Vab_Tr2D] -> Mux3/4
  Mux1/1 -> VsVpI_SH/1  "VaSec _VaPrim_IaPrim (pu)"
  [Iabc_SH] -> Selector/1
  [Vabc_B1] -> Selector1/1
  Selector1/1 -> Mux1/2
  Selector/1 -> Mux1/3
  Sum12/1 -> Mux1/1  "VaSec_SH"
  Demux/1 -> [VdcPM_SH], Sum2/1
  Demux/2 -> [VdcPM_SE], Sum3/1
  Sum2/1 -> Vdc_SH/1
  Sum3/1 -> Vdc_SE/1
  pp->pn1/1 -> Sum4/1
  Mux5/1 -> pp->pn1/1
  [Van_Tr1Yse] -> Mux5/1
  [Vab_Tr1Dse] -> Mux5/2
  [Van_Tr2Yse] -> Mux5/3
  [Vab_Tr2Dse] -> Mux5/4
  [Mag_rho_SE] -> Demux1/1
  Multimeter/1 -> Demux/1
  [MagVinj_SSSC] -> Mean/1
  Mean/1 -> Mux2/1

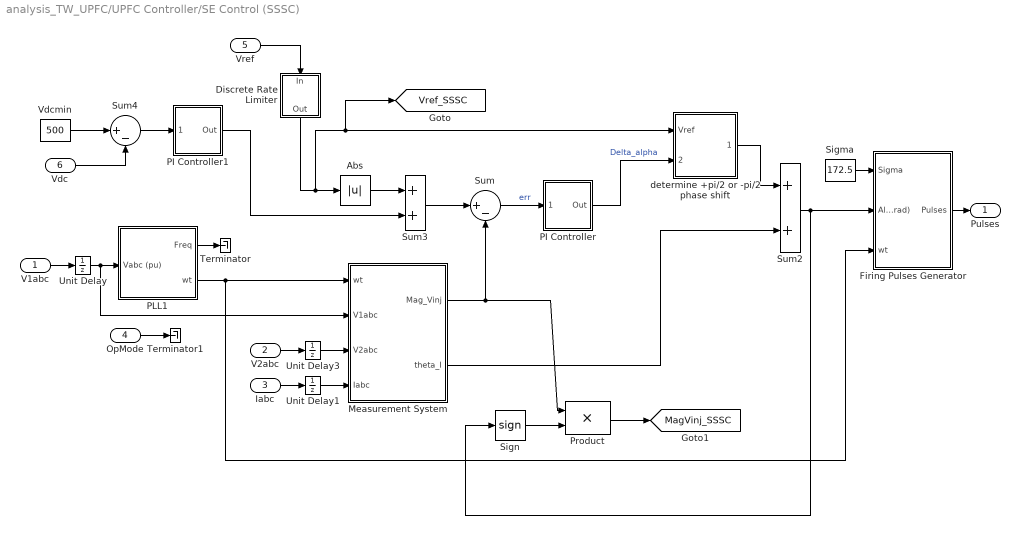
== system analysis_TW_UPFC/UPFC Controller/SE Control (SSSC) ==
  V1abc : Inport  PortDimensions=3
  V2abc : Inport  Port=2  PortDimensions=3
  Iabc : Inport  Port=3  PortDimensions=3
  OpMode : Inport  Port=4  PortDimensions=1
  Vref : Inport  Port=5  PortDimensions=1
  Vdc : Inport  Port=6  PortDimensions=1
  Abs : Abs  SaturateOnIntegerOverflow=on
  Discrete Rate Limiter : Subsystem  DialogController=POWERSYS.PowerSysDialog  mask(Discrete Rate Limiter){R=0.1*60/12, F=-0.1*60/12, Vinit=0.0, Ts=Ts}
      mask prompts: R "Rising slew rate:"; F "Falling slew rate:"; Vinit "Initial input:"; Ts "Sample time:"
      mask help: DISCRETE BLOCK : Limit rising and falling rates of signal
      mask init:
      | UpperLimit=R*Ts;
      | LowerLimit=F*Ts;
      | power_initmask();
      mask Help: This block is part of a subset of blocks in the Extras library that does not have documentation associated with it, other than the block mask description.
      mask Display: disp('Discrete\nRate\nLimiter')
  Firing Pulses Generator : Subsystem
  Measurement System : Subsystem
  PI Controller : Subsystem  DialogController=POWERSYS.PowerSysDialog  mask(Discrete PI Controller){Kp=2, Ki=100, Par_Limits=[1e6 -1e6], Init=0, Ts=Ts}
      mask prompts: Kp "Proportional gain (Kp):"; Ki "Integral gain (Ki):"; Par_Limits "Output limits: [ Upper   Lower ]"; Init "Output initial value:"; Ts "Sample time:"
      mask help: This block implements a discrete PI controller.
      mask init:
      | UpperLimit=Par_Limits(1);
      | LowerLimit=Par_Limits(2);
      | power_initmask();
      mask Help: This block is part of a subset of blocks in the Extras library that does not have documentation associated with it, other than the block mask description.
      mask Display: disp('PI');
  PI Controller1 : Subsystem  DialogController=POWERSYS.PowerSysDialog  mask(Discrete PI Controller){Kp=0.00005, Ki=0.002, Par_Limits=[0.02 0], Init=0, Ts=Ts}
      mask prompts: Kp "Proportional gain (Kp):"; Ki "Integral gain (Ki):"; Par_Limits "Output limits: [ Upper   Lower ]"; Init "Output initial value:"; Ts "Sample time:"
      mask help: This block implements a discrete PI controller.
      mask init:
      | UpperLimit=Par_Limits(1);
      | LowerLimit=Par_Limits(2);
      | power_initmask();
      mask Help: This block is part of a subset of blocks in the Extras library that does not have documentation associated with it, other than the block mask description.
      mask Display: disp('PI');
  PLL1 : Subsystem  mask(Discrete 3-phase PLL){Nstep=1, Par_Init=[0 60], ParK=[60 1400], Ts=Ts}
      mask prompts: Nstep "PLL timing correction (in number of time step)"; Par_Init "Initial inputs:[ Phase(degrees)   Frequency(Hz) ]"; ParK "Regulator gains [ Kp  Ki ]"; Ts "Sample time:"
      mask help:
      | This Phase Locked Loop (PLL) system can be used  to synchronize on a set of variable frequency, three-phase sinusoidal signals.
      |
      | Input 1: Vector containing the normalized
      |              three-phase signals [Va Vb Vc]
      | Output 1:  Measured frequency (Hz) = w/(2pi)
      | Output 2:  Ramp w.t   varying between  0 and 2*pi,
      | synchronized on zero crossings of the fundamental (positive-sequence) of phase A.
      | Output 3: Vector [sin(wt) cos(wt)]
      mask init:
      | Kp=ParK(1);
      | Ki=ParK(2);
      | Phase_Init=Par_Init(1);
      | Finit=Par_Init(2);
  Product : Product  SaturateOnIntegerOverflow=on  OutDataTypeStr=Inherit: Same as first input
  Sigma : Constant  Value=172.5
  Sign : Signum
  Sum : Sum  Inputs=|+-  SaturateOnIntegerOverflow=on
  Sum2 : Sum  SaturateOnIntegerOverflow=on
  Sum3 : Sum  SaturateOnIntegerOverflow=on
  Sum4 : Sum  Inputs=|+-  SaturateOnIntegerOverflow=on
  Terminator : Terminator
  Terminator1 : Terminator
  Unit Delay : UnitDelay  SampleTime=Ts
  Unit Delay1 : UnitDelay  SampleTime=Ts
  Unit Delay3 : UnitDelay  SampleTime=Ts
  Vdcmin : Constant  Value=500
  determine +pi/2 or -pi/2 phase shift : Subsystem
  Pulses : Outport
  tag scope: MagVinj_SSSC=global, Vref_SSSC=global
  wires:
  Discrete Rate Limiter/1(Out) -> Abs/1, determine +pi/2 or -pi/2 phase shift/1(Vref), [Vref_SSSC]
  PI Controller1/1(Out) -> Sum3/2
  Vdc/1 -> Sum4/2
  determine +pi/2 or -pi/2 phase shift/1(Alpha) -> Sum2/1
  PI Controller/1(Out) -> determine +pi/2 or -pi/2 phase shift/2(Delta_Alpha)  "Delta_alpha"
  Vdcmin/1 -> Sum4/1
  Sum4/1 -> PI Controller1/1(Error)
  Sum3/1 -> Sum/1
  Abs/1 -> Sum3/1
  Vref/1 -> Discrete Rate Limiter/1(In)
  Sum2/1 -> Firing Pulses Generator/2(Alpha(rad)), Sign/1
  Measurement System/2(theta_I) -> Sum2/2
  OpMode/1 -> Terminator1/1
  Sigma/1 -> Firing Pulses Generator/1(Sigma)
  Measurement System/1(Mag_Vinj) -> Sum/2, Product/1
  Sum/1 -> PI Controller/1(Error)  "err"
  Unit Delay3/1 -> Measurement System/3(V2abc)
  Unit Delay1/1 -> Measurement System/4(Iabc)
  PLL1/1(Freq) -> Terminator/1
  Unit Delay/1 -> PLL1/1(Vabc (pu)), Measurement System/2(V1abc)
  Firing Pulses Generator/1(Pulses) -> Pulses/1
  V1abc/1 -> Unit Delay/1
  V2abc/1 -> Unit Delay3/1
  Iabc/1 -> Unit Delay1/1
  PLL1/2(wt) -> Firing Pulses Generator/3(wt), Measurement System/1(wt)
  Product/1 -> [MagVinj_SSSC]
  Sign/1 -> Product/2

== system analysis_TW_UPFC/UPFC Controller/SE Control (UPFC) ==
  note: Pierre Giroux, Gilbert Sybille
      | Power System Simulation Laboratory
      | IREQ, Hydro-Quebc
  note: Series Controller
      | (48-pulse, 3-level Inverter)
  V1abc : Inport  PortDimensions=3
  V2abc : Inport  Port=2  PortDimensions=3
  I2abc : Inport  Port=3  PortDimensions=3
  VdcPM_SE : Inport  Port=4  PortDimensions=2
  OpMode : Inport  Port=5  PortDimensions=1
  PrefQref : Inport  Port=6  PortDimensions=2
  Constant2 : Constant  Value=0
  Current Regulators : Subsystem  mask(Current Regulators){Kp=Kp_Vseries, Ki=Ki_Vseries, Kd=0, TcD=0.2e-3, Par_Limits=[0.12 -0.12], Init=0, Ts=Ts}
      mask prompts: Kp "Proportional gain (Kp):"; Ki "Integral gain (Ki):"; Kd "Derivative gain (Kd):"; TcD "Time constant for derivative (s):"; Par_Limits "Output limits: [ Upper   Lower ]"; Init "Output initial value:"; Ts "Sample time:"
      mask help:
      | Sign convention:
      | Id positive(+) flowing into converter ==> Converter absorbing real power = P positive(+)
      | Iq negative(-) flowing into converter (inductive current) ==> Converter absorbing reactive power = Q positive(+)
  Firing Pulses Generator : Subsystem
  Mag/rho and sigma computation : Subsystem
  Measurement System : Subsystem
  Mux : Mux  Inputs=[2 2]
  Mux1 : Mux  Inputs=[2 2]
  PLL1 : Subsystem  mask(Discrete 3-phase PLL){Nstep=1, Par_Init=[0 60], ParK=[60 1400], Ts=Ts}
      mask prompts: Nstep "PLL timing correction (in number of time step)"; Par_Init "Initial inputs:[ Phase(degrees)   Frequency(Hz) ]"; ParK "Regulator gains [ Kp  Ki ]"; Ts "Sample time:"
      mask help:
      | This Phase Locked Loop (PLL) system can be used  to synchronize on a set of variable frequency, three-phase sinusoidal signals.
      |
      | Input 1: Vector containing the normalized
      |              three-phase signals [Va Vb Vc]
      | Output 1:  Measured frequency (Hz) = w/(2pi)
      | Output 2:  Ramp w.t   varying between  0 and 2*pi,
      | synchronized on zero crossings of the fundamental (positive-sequence) of phase A.
      | Output 3: Vector [sin(wt) cos(wt)]
      mask init:
      | Kp=ParK(1);
      | Ki=ParK(2);
      | Phase_Init=Par_Init(1);
      | Finit=Par_Init(2);
  Reference Computation : Subsystem
  Vd,Vq Selection (Auto/Man) and Limit Computation : Subsystem
  Pulses : Outport
  tag scope: IdqIdqref_SE=global, PQ_SE=global
  wires:
  Firing Pulses Generator/1(Pulses) -> Pulses/1
  V1abc/1 -> PLL1/1(Vabc (pu))
  V2abc/1 -> Measurement System/3(Vabc)
  PLL1/1(Freq) -> Measurement System/1(Freq)
  I2abc/1 -> Measurement System/4(Iabc)
  PLL1/2(wt) -> Measurement System/2(wt), Firing Pulses Generator/4(wt)
  Constant2/1 -> Firing Pulses Generator/2(D_Alpha)
  Mux1/1 -> [PQ_SE]
  Mux/1 -> [IdqIdqref_SE]
  PrefQref/1 -> Reference Computation/1(Pref_Qref), Mux1/2
  Reference Computation/1(Id*_Iq*) -> Current Regulators/1(Id_Iq_Ref), Mux/2
  Measurement System/1(PQ) -> Mux1/1
  Measurement System/2(Vd_Vq) -> Reference Computation/2(Vd_Vq)
  Measurement System/3(Id_Iq) -> Current Regulators/2(Id_Iq), Mux/1
  Current Regulators/1(VdVq*) -> Vd,Vq Selection (Auto/Man) and Limit Computation/1(VdVq*)
  VdcPM_SE/1 -> Mag/rho and sigma computation/2(VdcPM_SE)
  Vd,Vq Selection (Auto/Man) and Limit Computation/1(VdVq_inj) -> Mag/rho and sigma computation/1(VdVq)
  Mag/rho and sigma computation/1(Sigma) -> Firing Pulses Generator/1(Sigma)
  Mag/rho and sigma computation/2(rho) -> Firing Pulses Generator/3(Alpha)
  OpMode/1 -> Vd,Vq Selection (Auto/Man) and Limit Computation/2(OpMode)

== system analysis_TW_UPFC/UPFC Controller/SH Control (STATCOM) ==
  note: Pierre Giroux, Gilbert Sybille
      | Power System Simulation Laboratory
      | IREQ, Hydro-Quebc
  note: Shunt Controller
      | (48-pulse, 3-level Inverter)
  Vabc_In : Inport  PortDimensions=3
  Iabc_In : Inport  Port=2  PortDimensions=3
  VdcPN : Inport  Port=3  PortDimensions=2
  OpMode : Inport  Port=4  PortDimensions=1
  Qref : Inport  Port=5  PortDimensions=1
  Vref : Inport  Port=6  PortDimensions=1
  Current Regulator : Subsystem  mask(Discrete PI Controller){Kp=Kp_I, Ki=Ki_I, Par_Limits=[80 -80], Init=0, Ts=Ts}
      mask prompts: Kp "Proportional gain (Kp):"; Ki "Integral gain (Ki):"; Par_Limits "Output limits: [ Upper   Lower ]"; Init "Output initial value:"; Ts "Sample time:"
      mask help: This block implements a discrete PI controller.
      mask init:
      | UpperLimit=Par_Limits(1);
      | LowerLimit=Par_Limits(2);
  DC Balance Regulator : Subsystem
  Firing Pulses Generator : Subsystem
  Iq Limit Computation and Iqref Selection : Subsystem
  Measurement System : Subsystem
  Mux : Mux  Inputs=2
  Mux1 : Mux  Inputs=2
  PLL : Subsystem  mask(Discrete 3-phase PLL){Nstep=1, Par_Init=[0 60], ParK=[60 1400], Ts=Ts}
      mask prompts: Nstep "PLL timing correction (in number of time step)"; Par_Init "Initial inputs:[ Phase(degrees)   Frequency(Hz) ]"; ParK "Regulator gains [ Kp  Ki ]"; Ts "Sample time:"
      mask help:
      | This Phase Locked Loop (PLL) system can be used  to synchronize on a set of variable frequency, three-phase sinusoidal signals.
      |
      | Input 1: Vector containing the normalized
      |              three-phase signals [Va Vb Vc]
      | Output 1:  Measured frequency (Hz) = w/(2pi)
      | Output 2:  Ramp w.t   varying between  0 and 2*pi,
      | synchronized on zero crossings of the fundamental (positive-sequence) of phase A.
      | Output 3: Vector [sin(wt) cos(wt)]
      mask init:
      | Kp=ParK(1);
      | Ki=ParK(2);
      | Phase_Init=Par_Init(1);
      | Finit=Par_Init(2);
  Qref (pu)1 : Constant  Value=Iqref1
  Sigma (deg) : Constant  Value=180-7.5
  Unit Delay3 : UnitDelay  SampleTime=Ts
  Voltage Regulator : Subsystem  mask(Discrete PI Controller){Droop=Droop, Kp=Kp_V, Ki=Ki_V, Par_Limits=[1 -1], Init=0, Ts=Ts}
      mask prompts: Droop "Droop (pu/100MVA):"; Kp "Proportional gain (Kp):"; Ki "Integral gain (Ki):"; Par_Limits "Output limits: [ Upper   Lower ]"; Init "Output initial value:"; Ts "Sample time:"
      mask help: This block implements a discrete PI controller.
      mask init:
      | UpperLimit=Par_Limits(1);
      | LowerLimit=Par_Limits(2);
  Pulses : Outport
  tag scope: IqIqref_SH=global, PQ_SH=global, VmesVref_SH=global, alpha_SH=global
  wires:
  Iabc_In/1 -> Measurement System/2(Iabc)
  Firing Pulses Generator/1(Pulses) -> Pulses/1
  VdcPN/1 -> DC Balance Regulator/2(+/-Vdc/2)
  Mux/1 -> [VmesVref_SH]
  Unit Delay3/1 -> DC Balance Regulator/1(Iq_avg)
  Measurement System/4(Iq_avg) -> Unit Delay3/1
  Vabc_In/1 -> Measurement System/1(Vabc), PLL/1(Vabc (pu))
  PLL/2(wt) -> Measurement System/4(wt), Firing Pulses Generator/3(wt)  "wt"
  PLL/1(Freq) -> Measurement System/3(Freq)
  OpMode/1 -> Iq Limit Computation and Iqref Selection/5(OpMode)
  Voltage Regulator/1(Iqref) -> Iq Limit Computation and Iqref Selection/2(Iqref(Auto))
  Measurement System/2(PQ) -> [PQ_SH]
  Measurement System/1(Vmes) -> Mux/1, Iq Limit Computation and Iqref Selection/1(Vmes), Voltage Regulator/2(Vmes)
  Qref (pu)1/1 -> Iq Limit Computation and Iqref Selection/4(Iqref1)
  Measurement System/3(Iq) -> Current Regulator/2(Iq), Mux1/1
  Measurement System/5(Id) -> Iq Limit Computation and Iqref Selection/6(Id)
  Vref/1 -> Voltage Regulator/1(Vref), Mux/2
  Iq Limit Computation and Iqref Selection/1(Iqref) -> Current Regulator/1(Iq_Ref), Mux1/2
  Mux1/1 -> [IqIqref_SH]
  Sigma (deg)/1 -> Firing Pulses Generator/2(Sigma)
  DC Balance Regulator/1(D_Alpha) -> Firing Pulses Generator/4(D_Alpha)
  Current Regulator/1(Alpha) -> Firing Pulses Generator/1(Alpha), [alpha_SH]
  Qref/1 -> Iq Limit Computation and Iqref Selection/3(Qref1)

== system analysis_TW_UPFC/Subsystem4/Data Acquisition/Power Computation ==
  Mux4 : Mux  Inputs=6
  Power (Positive-Sequence) : powerlib_meascontrol/Measurements/Power (Positive-Sequence)  Freq=60  Vinit=[1, 0]  Iinit=[6.575 3.94]  Ts=Ts
      settings: SourceProductName=Simscape Power Systems  SourceProductBaseCode=PS
  Power (Positive-Sequence)1 : powerlib_meascontrol/Measurements/Power (Positive-Sequence)  Freq=60  Vinit=[1, 0]  Iinit=[8.72 4.1]  Ts=Ts
      settings: SourceProductName=Simscape Power Systems  SourceProductBaseCode=PS
  Power (Positive-Sequence)2 : powerlib_meascontrol/Measurements/Power (Positive-Sequence)  Freq=60  Vinit=[1, 0]  Iinit=[9.605 0.36]  Ts=Ts
      settings: SourceProductName=Simscape Power Systems  SourceProductBaseCode=PS
  Selector2 : Selector  InputPortWidth=6  IndexOptions=Index vector (dialog)  Indices=[1 3 5]  OutputSizes=1
  Selector3 : Selector  InputPortWidth=6  IndexOptions=Index vector (dialog)  Indices=[1 3 5]+1  OutputSizes=1
  Sum1 : Sum  Inputs=+--  SaturateOnIntegerOverflow=on  InputSameDT=on  OutDataTypeStr=Inherit: Same as first input
  V>pu2 : Gain  Gain=2/3*100  SaturateOnIntegerOverflow=on  OutDataTypeStr=Inherit: Same as input  ParamDataTypeStr=Inherit: Same as input
  Ps : Outport
  Qs : Outport  Port=2
  wires:
  [Iabc_B1] -> Sum1/1
  [Iabc_SE] -> Sum1/2
  [Iabc_SH] -> Sum1/3
  [Vabc_B1] -> Power (Positive-Sequence)2/1
  Sum1/1 -> Power (Positive-Sequence)2/2
  [Vabc_B2] -> Power (Positive-Sequence)1/1
  [Iabc_B2] -> Power (Positive-Sequence)1/2
  [Vabc_B3] -> Power (Positive-Sequence)/1
  [Iabc_B3] -> Power (Positive-Sequence)/2
  Mux4/1 -> V>pu2/1
  V>pu2/1 -> Selector2/1, Selector3/1
  Selector2/1 -> Ps/1
  Selector3/1 -> Qs/1
  Power (Positive-Sequence)/2 -> Mux4/6
  Power (Positive-Sequence)/1 -> Mux4/5
  Power (Positive-Sequence)1/2 -> Mux4/4
  Power (Positive-Sequence)1/1 -> Mux4/3
  Power (Positive-Sequence)2/2 -> Mux4/2
  Power (Positive-Sequence)2/1 -> Mux4/1

== system analysis_TW_UPFC/UPFC Controller/SE Control (SSSC)/Discrete Rate Limiter ==
  note: Beat Ronner
      | ABB Industrie AG
      | Turgi, Switzerland
  note: Delta(u)
  In : Inport
  Saturation : Saturate  UpperLimit=UpperLimit  LowerLimit=LowerLimit
  Sum : Sum  Inputs=|++  SaturateOnIntegerOverflow=on  InputSameDT=on  OutDataTypeStr=Inherit: Same as first input
  Sum1 : Sum  Inputs=|+-  SaturateOnIntegerOverflow=on  InputSameDT=on  OutDataTypeStr=Inherit: Same as first input
  Unit Delay : UnitDelay  InitialCondition=Vinit  SampleTime=Ts
  Out : Outport
  wires:
  Unit Delay/1 -> Sum/2, Sum1/2  "y-1"
  Sum/1 -> Unit Delay/1, Out/1  "y"
  Saturation/1 -> Sum/1  "Delta(u)_limit"
  Sum1/1 -> Saturation/1
  In/1 -> Sum1/1  "u"
